simulink model "Lab2_massspringdamper"  (R2018b)
settings: Solver=FixedStepAuto  StartTime=0.0  StopTime=10.0  FixedStep=0.0001  RelTol=1e-3
values from neighbouring files (symbols this model uses):
  B = 25    [Lab2_Mass_Spring_Damper.m]
  K = 16    [Lab2_Mass_Spring_Damper.m]
  M = 20    [Lab2_Mass_Spring_Damper.m]
settings Model: NumberOfSteps=5  Creator=student  LastModifiedBy=Harsh

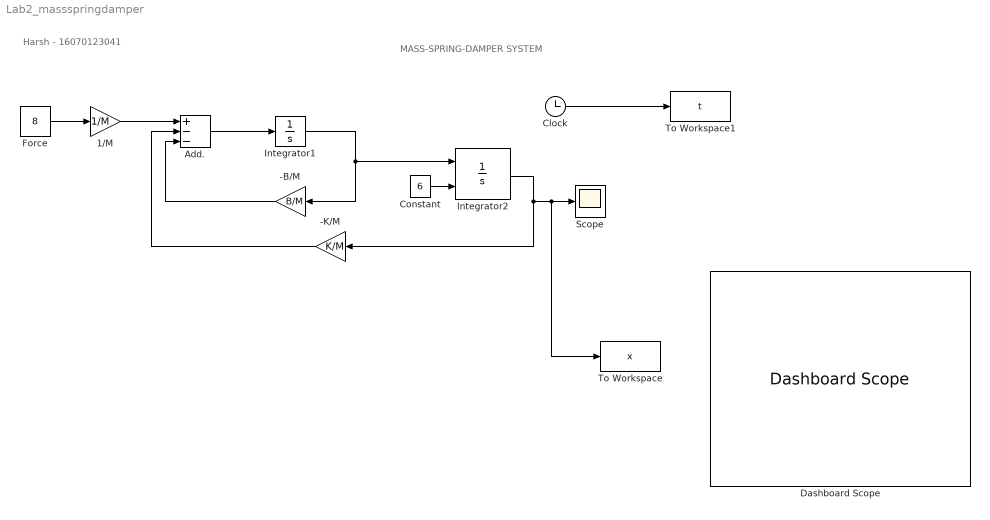
== system Lab2_massspringdamper ==
  note: Harsh - 16070123041
  note: MASS-SPRING-DAMPER SYSTEM
  -B/M : Gain  Gain=B/M
  -K/M : Gain  Gain=K/M
  1/M : Gain  Gain=1/M
  Add. : Sum  Inputs=+--
  Clock : Clock
  Constant : Constant  Value=6
  Dashboard Scope : DashboardScope  WebBlockId=52
  Force : Constant  Value=8
  Integrator1 : Integrator
  Integrator2 : Integrator  InitialConditionSource=external  InitialCondition=5
  Scope : Scope
  To Workspace : ToWorkspace  VariableName=x  SampleTime=-1
  To Workspace1 : ToWorkspace  VariableName=t  SampleTime=-1
  wires:
  Integrator1/1 -> -B/M/1, Integrator2/1
  Add./1 -> Integrator1/1
  Clock/1 -> To Workspace1/1
  Constant/1 -> Integrator2/2
  Force/1 -> 1/M/1
  Integrator2/1 -> -K/M/1, To Workspace/1, Scope/1
  1/M/1 -> Add./1
  -B/M/1 -> Add./3
  -K/M/1 -> Add./2
